simulink model "part1_Simulation1"  (R2014b)
settings: Solver=VariableStepAuto  StartTime=0.0  StopTime=10  RelTol=1e-3
values from neighbouring files (symbols this model uses):
  getPos = [0; 0; 1]    [init_Sim1.m]    (also in init_Sim3.m; init_Sim4.m)
  getVel = [0;1;0]    [init_Sim1.m]    (also in init_Sim3.m; init_Sim4.m)
  Kd = 7*[M3(1)*Omega 0 0; 0 M3(2,2)*Omega 0; 0 0 20*M(3,3)*Omega]    [init_Sim1.m]    (also in init_Sim3.m; init_Sim4.m)
  Ki = 100*(omega/10)*[M3(1)*omega^2 0 0;0 M3(2,2)*omega^2 0; 0 0 M3(3,3)*omega^2 ]*2    [init_Sim1.m]    (also in init_Sim3.m; init_Sim4.m)
  Kp = 50*[M3(1)*omega^2 0 0;0 M3(2,2)*omega^2 0; 0 0 15*M3(3,3)*omega^2 ]    [init_Sim1.m]    (also in init_Sim3.m; init_Sim4.m)
  Omega = 2*damping*omega    [init_Sim1.m]    (also in init_Sim3.m; init_Sim4.m)
  omega = omegab/sqrt(1-2*damping^2+sqrt(4*damping^4-4*damping^2+2))    [init_Sim1.m]    (also in init_Sim3.m; init_Sim4.m)
  phi = 3/8    (= 0.375)    [init_Sim1.m]    (also in init_Sim3.m)
  ref = [50;0;0]    [init_Sim1.m]    (also in init_Sim3.m = [10 10 -pi/2]; init_Sim4.m = [0;0;0])
  Vc = 1    [init_Sim1.m]    (also in init_Sim3.m; init_Sim4.m)
undefined symbols (not defined in the file or in its folder): Hoerner, vessel
libraries: simulink x2, marine_hydro x1
settings Model: Creator=jonbjor  LastModifiedBy=Karianne
settings DataIOCC: LimitDataPoints=off  SaveFormat=Dataset
settings OptimizationCC: UseDivisionForNetSlopeComputation=off  LifeSpan=auto  SimCompilerOptimization=off
settings DebuggingCC: SolverPrmCheckMsg=none  FcnCallInpInsideContextMsg=error  FrameProcessingCompatibilityMsg=error  SFUnexpectedBacktrackingDiag=error  SFNoUnconditionalDefaultTransitionDiag=error
settings HardwareCC: ProdBitPerPointer=64  ProdLargestAtomicFloat=Float  ProdIntDivRoundTo=Zero  ProdEndianess=LittleEndian  ProdWordSize=64  ProdHWDeviceType=Intel->x86-64 (Windows64)
settings ModelReferenceCC: PropagateSignalLabelsOutOfModel=on
settings RTWCC: RTWCompilerOptimization=off
settings GRTTargetCC: TargetLangStandard=C99 (ISO)  GeneratePreprocessorConditionals=Use local settings

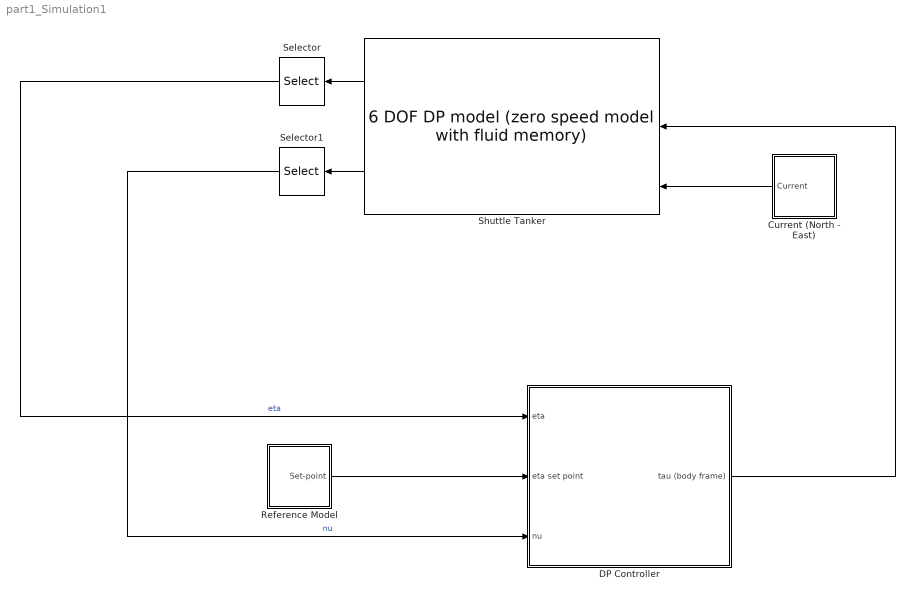
== system part1_Simulation1 ==
  Current (North - East) : Subsystem
  DP Controller : Subsystem
  Reference Model : Subsystem
  Selector : Selector  InputPortWidth=6  Indices=[1 2 6]
  Selector1 : Selector  InputPortWidth=6  Indices=[1 2 6]
  Shuttle Tanker : marine_hydro/Hydro Library/6 DOF DP model  (zero speed model with fluid memory)  ABC=vesselABC  rho=1025  Axc=0.9*vessel.main.T*vessel.main.B  Ayc=0.9*vessel.main.T*vessel.main.Lpp  CX=1  CY_2D=Hoerner(vessel.main.B,vessel.main.T)  Bv=vessel.Bv
      link override "Integrator1 ": InitialCondition=nu0
      link override Integrator2: InitialCondition=eta0
  wires:
  DP Controller/1(tau (body frame)) -> Shuttle Tanker/2
  Shuttle Tanker/1 -> Selector/1
  Shuttle Tanker/2 -> Selector1/1
  Reference Model/1(Set-point) -> DP Controller/2(eta set point)
  Selector1/1 -> DP Controller/3(nu)  "nu"
  Selector/1 -> DP Controller/1(eta)  "eta"
  Current (North - East)/1(Current) -> Shuttle Tanker/3

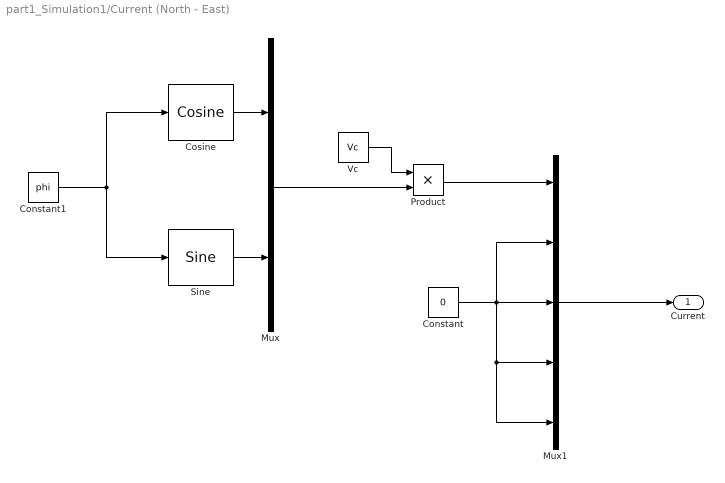
== system part1_Simulation1/Current (North - East) ==
  Constant : Constant  Value=0
  Constant1 : Constant  Value=phi
  Cosine : simulink/Lookup Tables/Cosine  Formula=cos(2*pi*u)  NumDataPoints=(2^5)+1  OutputWordLength=16  InternalRulePriority=Speed
  Mux : Mux  Inputs=2
  Mux1 : Mux  Inputs=5
  Product : Product  SaturateOnIntegerOverflow=off  RndMeth=Floor  InputSameDT=off  OutDataTypeStr=Inherit: Inherit via internal rule
  Sine : simulink/Lookup Tables/Sine  Formula=sin(2*pi*u)  NumDataPoints=(2^5)+1  OutputWordLength=16  InternalRulePriority=Speed
  Vc : Constant  Value=Vc
  Current : Outport
  wires:
  Sine/1 -> Mux/2
  Mux/1 -> Product/2
  Cosine/1 -> Mux/1
  Product/1 -> Mux1/1
  Constant/1 -> Mux1/5, Mux1/4, Mux1/3, Mux1/2
  Mux1/1 -> Current/1
  Vc/1 -> Product/1
  Constant1/1 -> Sine/1, Cosine/1

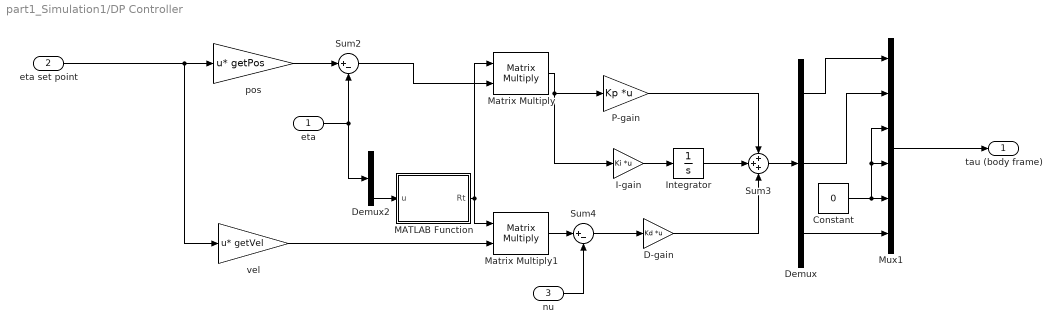
== system part1_Simulation1/DP Controller ==
  eta : Inport
  eta set point : Inport  Port=2
  nu : Inport  Port=3
  Constant : Constant  Value=0
  D-gain : Gain  Gain=Kd  Multiplication=Matrix(K*u)  SaturateOnIntegerOverflow=off  OutDataTypeStr=Inherit: Inherit via internal rule  ParamDataTypeStr=Inherit: Inherit via internal rule
  Demux : Demux  Outputs=3
  Demux2 : Demux  Outputs=3
  I-gain : Gain  Gain=Ki  Multiplication=Matrix(K*u)  SaturateOnIntegerOverflow=off  OutDataTypeStr=Inherit: Inherit via internal rule  ParamDataTypeStr=Inherit: Inherit via internal rule
  Integrator : Integrator
  MATLAB Function : MATLAB Function  TreatAsAtomicUnit=on
  Matrix Multiply : Product  Multiplication=Matrix(*)  SaturateOnIntegerOverflow=off  RndMeth=Floor  InputSameDT=off  OutDataTypeStr=Inherit: Inherit via internal rule
  Matrix Multiply1 : Product  Multiplication=Matrix(*)  SaturateOnIntegerOverflow=off  RndMeth=Floor  InputSameDT=off  OutDataTypeStr=Inherit: Inherit via internal rule
  Mux1 : Mux  Inputs=6
  P-gain : Gain  Gain=Kp  Multiplication=Matrix(K*u)  SaturateOnIntegerOverflow=off  OutDataTypeStr=Inherit: Inherit via internal rule  ParamDataTypeStr=Inherit: Inherit via internal rule
  Sum2 : Sum  Inputs=|+-  SaturateOnIntegerOverflow=off  InputSameDT=off  OutDataTypeStr=Inherit: Inherit via internal rule
  Sum3 : Sum  Inputs=+++  SaturateOnIntegerOverflow=off  InputSameDT=off  OutDataTypeStr=Inherit: Inherit via internal rule
  Sum4 : Sum  Inputs=|+-  SaturateOnIntegerOverflow=off  InputSameDT=off  OutDataTypeStr=Inherit: Inherit via internal rule
  pos : Gain  Gain=getPos  Multiplication=Matrix(u*K)  SaturateOnIntegerOverflow=off  OutDataTypeStr=Inherit: Inherit via internal rule  ParamDataTypeStr=Inherit: Inherit via internal rule
  vel : Gain  Gain=getVel  Multiplication=Matrix(u*K)  SaturateOnIntegerOverflow=off  OutDataTypeStr=Inherit: Inherit via internal rule  ParamDataTypeStr=Inherit: Inherit via internal rule
  tau (body frame) : Outport
  wires:
  eta/1 -> Demux2/1, Sum2/2
  I-gain/1 -> Integrator/1
  Sum3/1 -> Demux/1
  Demux/1 -> Mux1/1
  Demux/2 -> Mux1/2
  Demux/3 -> Mux1/6
  Constant/1 -> Mux1/4, Mux1/3, Mux1/5
  Mux1/1 -> tau (body frame)/1
  Demux2/3 -> MATLAB Function/1(u)
  nu/1 -> Sum4/2
  Matrix Multiply1/1 -> Sum4/1
  Sum4/1 -> D-gain/1
  P-gain/1 -> Sum3/1
  Matrix Multiply/1 -> I-gain/1, P-gain/1
  Integrator/1 -> Sum3/2
  D-gain/1 -> Sum3/3
  Sum2/1 -> Matrix Multiply/2
  MATLAB Function/1(Rt) -> Matrix Multiply/1, Matrix Multiply1/1
  vel/1 -> Matrix Multiply1/2
  eta set point/1 -> vel/1, pos/1
  pos/1 -> Sum2/1

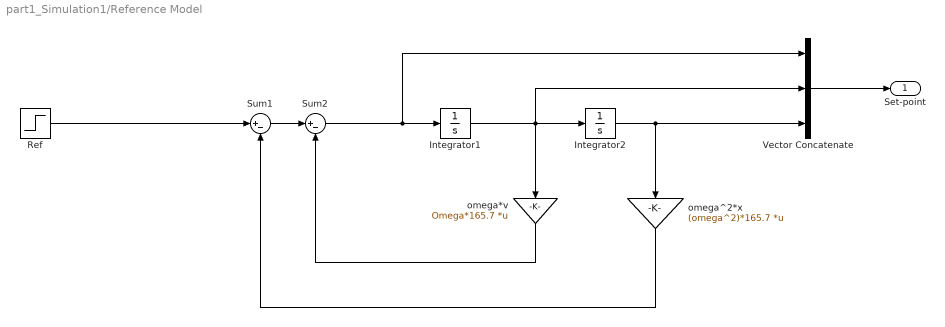
== system part1_Simulation1/Reference Model ==
  Integrator1 : Integrator
  Integrator2 : Integrator
  Ref : Step  Time=50  After=ref  SampleTime=0
  Sum1 : Sum  Inputs=|+-  SaturateOnIntegerOverflow=off  InputSameDT=off  OutDataTypeStr=Inherit: Inherit via internal rule
  Sum2 : Sum  Inputs=|+-  SaturateOnIntegerOverflow=off  InputSameDT=off  OutDataTypeStr=Inherit: Inherit via internal rule
  Vector Concatenate : Concatenate  NumInputs=3  Mode=Multidimensional array  ConcatenateDimension=2
  omega*v : Gain  Gain=Omega*165.7  Multiplication=Matrix(K*u)  SaturateOnIntegerOverflow=off  OutDataTypeStr=Inherit: Inherit via internal rule  ParamDataTypeStr=Inherit: Inherit via internal rule
  omega^2*x : Gain  Gain=(omega^2)*165.7  Multiplication=Matrix(K*u)  SaturateOnIntegerOverflow=off  OutDataTypeStr=Inherit: Inherit via internal rule  ParamDataTypeStr=Inherit: Inherit via internal rule
  Set-point : Outport
  wires:
  omega^2*x/1 -> Sum1/2
  Vector Concatenate/1 -> Set-point/1
  Sum1/1 -> Sum2/1
  omega*v/1 -> Sum2/2
  Integrator2/1 -> Vector Concatenate/3, omega^2*x/1
  Integrator1/1 -> Vector Concatenate/2, omega*v/1, Integrator2/1
  Sum2/1 -> Vector Concatenate/1, Integrator1/1
  Ref/1 -> Sum1/1

== matlab function part1_Simulation1/DP Controller/MATLAB Function ==
  data: u input; Rt output
function Rt = fcn(u)

R=[cos(u) -sin(u) 0; sin(u) cos(u) 0; 0 0 1];
Rt=transpose(R);

end
